simulink model "DYC_controller"  (R2018b)
settings: Solver=FixedStepAuto  StartTime=0.0  StopTime=inf  FixedStep=Ts  RelTol=1e-3  EnableMultiTasking=on
values from neighbouring files (symbols this model uses):
  A_vte = [1 0 -2*Ts*m_s/WB*(l_r*h_rc_f/w1+l_f*h_rc_r/w2) 0 -2*Ts*(K_f/w1+K_r/w2) ... (first row only)    [main.m]
  A_vte_p2 = [1 0 0 0 0 -Ts * m * hc / 2 / WB 0 -Ts * l_r * m * hc / WB / w1 ... (first row only)    [main.m]
  b1 = ones(4,1)/R    [main.m]
  boundary = 3000    [main.m]
  C_vte = [0 1 0 g 0 ... (first row only)    [main.m]
  C_vte_p2 = [1, -1, 1, -1, 0, 0, 0, 0 ... (first row only)    [main.m]
  eta = 0    [main.m]
  F_z1_s = l_r * m * g / 2 / WB    (= 9.45353456158)    [main.m]
  F_z2_s = F_z1_s    (= 9.45353456158)    [main.m]
  F_z3_s = l_f * m * g / 2 / WB    (= 9.11094809852)    [main.m]
  F_z4_s = F_z3_s    (= 9.11094809852)    [main.m]
  g = 9.81    [main.m]
  h_rc_f = 0.00    (= 0)    [main.m]
  h_rc_r = 0.00    (= 0)    [main.m]
  hc = 0.0751    [main.m]
  J = 0.9    [main.m]
  k1 = 2000    [main.m]
  k2 = 1000    [main.m]
  K_f = K_lin*l_cs^2*cos(phi*pi/180)    [main.m]
  K_r = K_lin*l_cs^2*cos(phi*pi/180)    [main.m]
  Kd = 0    [main.m]
  Ki = 75    [main.m]
  Kp = 600    [main.m]
  l_f = 0.1968    [main.m]
  l_r = 0.2042    [main.m]
  m = 3.832    [main.m]
  m_s = 0.9*m    (= 3.4488)    [main.m]
  mu = 0.8    [main.m]
  Protean_PD18_motormap = [2.92104016907 601.978033502 650.789692516 685.109940533 725.756581133 754.659963437 780.850883334 807.9513301 837.761936672 868.484372712 893.788791739 922.70944354 ... (50 elements, 25x2)]    [Protean_PD18_motormap.mat]
  Q_lat_process = 1E0*[var_r^2  0 0 0 0 0 0 0 0 ... (first row only)    [main.m]
  Q_lat_sensor = 1E-2*[var_r_s^2 0 0 0 ... (first row only)    [main.m]
  Q_meas_susp_p1 = [var_ay_m_p^2 0 0 0 ... (first row only)    [main.m]
  Q_meas_susp_p2 = [var_del_Fz^2 0 0 0 0 ... (first row only)    [main.m]
  R = 0.055    [main.m]
  Ts = 0.015    [main.m]
  V_x0 = (1000/3600)*V_x0    (= 11.1111111111)    [main.m]
  w1 = 0.2824    [main.m]
  w2 = 2.929    [main.m]
  WB = 0.406    [main.m]
undefined symbols (not defined in the file or in its folder): C_lf, C_lr, DiscIntNeverNeededParam, Discrete, t_e, Time
libraries: raspberrypilib x24, hdlsllib x21, simulink x17, discretizing x2, ctrlSharedLib x2, sharedTrackingLibrary x1
(part 2 of 3)

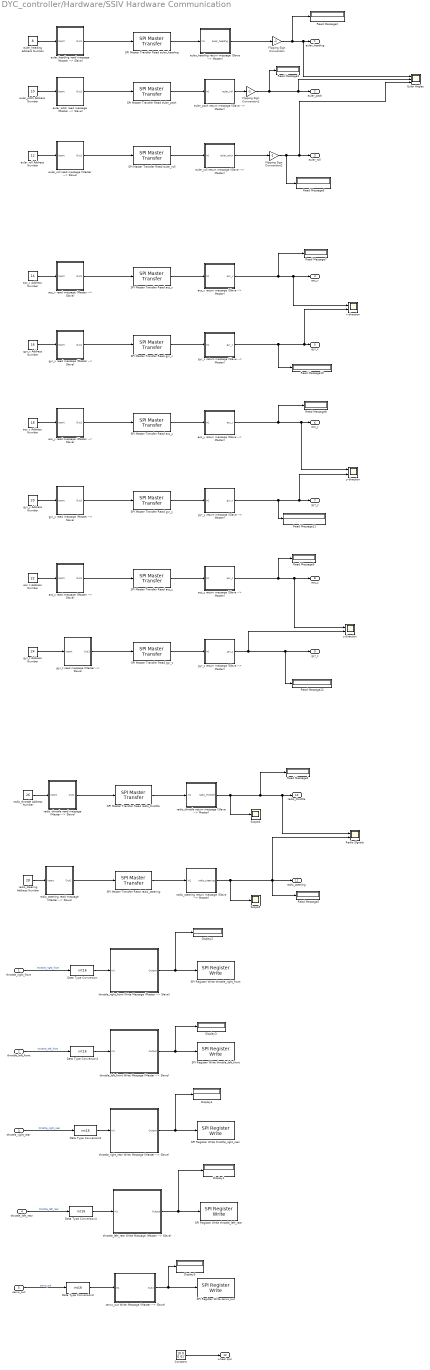
== system DYC_controller/Hardware/SSIV Hardware Communication ==
  throttle_right_front : Inport
  throttle_left_front : Inport  Port=2
  throttle_right_rear : Inport  Port=3
  throttle_left_rear : Inport  Port=4
  servo_out : Inport  Port=5
  Constant : Constant  Value=[0 0 0 0]'
  Data Type Conversion{,1..4} (5 alike) : DataTypeConversion  OutDataTypeStr=int16  RndMeth=Nearest
  Display{1..5} (5 alike) : Display
      settings: Format=decimal (Stored Integer)
  Euler Angles : Scope  NumInputPorts=3
  Flipping Sign Convention : Gain  Gain=-1
  Flipping Sign Convention1 : Gain  Gain=-1
  Flipping Sign Convention2 : Gain  Gain=-1
  Radio SIgnals : Scope  NumInputPorts=2
  Read Message{2..12} (11 alike) : Display
      settings: Format=decimal (Stored Integer)
  SPI Master Transfer Read acc_x : raspberrypilib/SPI Master Transfer  BoardProperty=Pi 3 Model B  SPIModule=uint32(0)  Mode=Master  BusSpeed=1000000  Pin=SPI0_CE1  FirstBitToTransfer=Most significant bit (MSB)  ClockMode=0  BlockFunction=Transfer  RegisterAddress=0  OutputDataType=int8  OutputDataLength=1
      settings: SourceProductName=Simulink Support Package for Raspberry Pi Hardware  SourceProductBaseCode=RASPPI
  SPI Master Transfer Read acc_y : raspberrypilib/SPI Master Transfer  BoardProperty=Pi 3 Model B  SPIModule=uint32(0)  Mode=Master  BusSpeed=1000000  Pin=SPI0_CE1  FirstBitToTransfer=Most significant bit (MSB)  ClockMode=0  BlockFunction=Transfer  RegisterAddress=0  OutputDataType=int8  OutputDataLength=1
      settings: SourceProductName=Simulink Support Package for Raspberry Pi Hardware  SourceProductBaseCode=RASPPI
  SPI Master Transfer Read acc_z : raspberrypilib/SPI Master Transfer  BoardProperty=Pi 3 Model B  SPIModule=uint32(0)  Mode=Master  BusSpeed=1000000  Pin=SPI0_CE1  FirstBitToTransfer=Most significant bit (MSB)  ClockMode=0  BlockFunction=Transfer  RegisterAddress=0  OutputDataType=int8  OutputDataLength=1
      settings: SourceProductName=Simulink Support Package for Raspberry Pi Hardware  SourceProductBaseCode=RASPPI
  SPI Master Transfer Read euler_heading : raspberrypilib/SPI Master Transfer  BoardProperty=Pi 3 Model B  SPIModule=uint32(0)  Mode=Master  BusSpeed=1000000  Pin=SPI0_CE1  FirstBitToTransfer=Most significant bit (MSB)  ClockMode=0  BlockFunction=Transfer  RegisterAddress=0  OutputDataType=int8  OutputDataLength=1
      settings: SourceProductName=Simulink Support Package for Raspberry Pi Hardware  SourceProductBaseCode=RASPPI
  SPI Master Transfer Read euler_pitch : raspberrypilib/SPI Master Transfer  BoardProperty=Pi 3 Model B  SPIModule=uint32(0)  Mode=Master  BusSpeed=1000000  Pin=SPI0_CE1  FirstBitToTransfer=Most significant bit (MSB)  ClockMode=0  BlockFunction=Transfer  RegisterAddress=0  OutputDataType=int8  OutputDataLength=1
      settings: SourceProductName=Simulink Support Package for Raspberry Pi Hardware  SourceProductBaseCode=RASPPI
  SPI Master Transfer Read euler_roll : raspberrypilib/SPI Master Transfer  BoardProperty=Pi 3 Model B  SPIModule=uint32(0)  Mode=Master  BusSpeed=1000000  Pin=SPI0_CE1  FirstBitToTransfer=Most significant bit (MSB)  ClockMode=0  BlockFunction=Transfer  RegisterAddress=0  OutputDataType=int8  OutputDataLength=1
      settings: SourceProductName=Simulink Support Package for Raspberry Pi Hardware  SourceProductBaseCode=RASPPI
  SPI Master Transfer Read gyr_x : raspberrypilib/SPI Master Transfer  BoardProperty=Pi 3 Model B  SPIModule=uint32(0)  Mode=Master  BusSpeed=1000000  Pin=SPI0_CE1  FirstBitToTransfer=Most significant bit (MSB)  ClockMode=0  BlockFunction=Transfer  RegisterAddress=0  OutputDataType=int8  OutputDataLength=1
      settings: SourceProductName=Simulink Support Package for Raspberry Pi Hardware  SourceProductBaseCode=RASPPI
  SPI Master Transfer Read gyr_y : raspberrypilib/SPI Master Transfer  BoardProperty=Pi 3 Model B  SPIModule=uint32(0)  Mode=Master  BusSpeed=1000000  Pin=SPI0_CE1  FirstBitToTransfer=Most significant bit (MSB)  ClockMode=0  BlockFunction=Transfer  RegisterAddress=0  OutputDataType=int8  OutputDataLength=1
      settings: SourceProductName=Simulink Support Package for Raspberry Pi Hardware  SourceProductBaseCode=RASPPI
  SPI Master Transfer Read gyr_z : raspberrypilib/SPI Master Transfer  BoardProperty=Pi 3 Model B  SPIModule=uint32(0)  Mode=Master  BusSpeed=1000000  Pin=SPI0_CE1  FirstBitToTransfer=Most significant bit (MSB)  ClockMode=0  BlockFunction=Transfer  RegisterAddress=0  OutputDataType=int8  OutputDataLength=1
      settings: SourceProductName=Simulink Support Package for Raspberry Pi Hardware  SourceProductBaseCode=RASPPI
  SPI Master Transfer Read radio_steering : raspberrypilib/SPI Master Transfer  BoardProperty=Pi 3 Model B  SPIModule=uint32(0)  Mode=Master  BusSpeed=1000000  Pin=SPI0_CE1  FirstBitToTransfer=Most significant bit (MSB)  ClockMode=0  BlockFunction=Transfer  RegisterAddress=0  OutputDataType=int8  OutputDataLength=1
      settings: SourceProductName=Simulink Support Package for Raspberry Pi Hardware  SourceProductBaseCode=RASPPI
  SPI Master Transfer Read radio_throttle : raspberrypilib/SPI Master Transfer  BoardProperty=Pi 3 Model B  SPIModule=uint32(0)  Mode=Master  BusSpeed=1000000  Pin=SPI0_CE1  FirstBitToTransfer=Most significant bit (MSB)  ClockMode=0  BlockFunction=Transfer  RegisterAddress=0  OutputDataType=int8  OutputDataLength=1
      settings: SourceProductName=Simulink Support Package for Raspberry Pi Hardware  SourceProductBaseCode=RASPPI
  "SPI Register Write servo_out " : raspberrypilib/SPI Register Write  BoardProperty=Pi 3 Model B  SPIModule=uint32(0)  Mode=Master  BusSpeed=1000000  Pin=SPI0_CE1  FirstBitToTransfer=Most significant bit (MSB)  ClockMode=0  BlockFunction=Write  RegisterAddress=38  OutputDataType=int8  OutputDataLength=1
      settings: SourceProductName=Simulink Support Package for Raspberry Pi Hardware  SourceProductBaseCode=RASPPI
  SPI Register Write throttle_left_front : raspberrypilib/SPI Register Write  BoardProperty=Pi 3 Model B  SPIModule=uint32(0)  Mode=Master  BusSpeed=1000000  Pin=SPI0_CE1  FirstBitToTransfer=Most significant bit (MSB)  ClockMode=0  BlockFunction=Write  RegisterAddress=32  OutputDataType=int8  OutputDataLength=1
      settings: SourceProductName=Simulink Support Package for Raspberry Pi Hardware  SourceProductBaseCode=RASPPI
  SPI Register Write throttle_left_rear : raspberrypilib/SPI Register Write  BoardProperty=Pi 3 Model B  SPIModule=uint32(0)  Mode=Master  BusSpeed=1000000  Pin=SPI0_CE1  FirstBitToTransfer=Most significant bit (MSB)  ClockMode=0  BlockFunction=Write  RegisterAddress=36  OutputDataType=int8  OutputDataLength=1
      settings: SourceProductName=Simulink Support Package for Raspberry Pi Hardware  SourceProductBaseCode=RASPPI
  SPI Register Write throttle_right_front : raspberrypilib/SPI Register Write  BoardProperty=Pi 3 Model B  SPIModule=uint32(0)  Mode=Master  BusSpeed=1000000  Pin=SPI0_CE1  FirstBitToTransfer=Most significant bit (MSB)  ClockMode=0  BlockFunction=Write  RegisterAddress=30  OutputDataType=int8  OutputDataLength=1
      settings: SourceProductName=Simulink Support Package for Raspberry Pi Hardware  SourceProductBaseCode=RASPPI
  SPI Register Write throttle_right_rear : raspberrypilib/SPI Register Write  BoardProperty=Pi 3 Model B  SPIModule=uint32(0)  Mode=Master  BusSpeed=1000000  Pin=SPI0_CE1  FirstBitToTransfer=Most significant bit (MSB)  ClockMode=0  BlockFunction=Write  RegisterAddress=34  OutputDataType=int8  OutputDataLength=1
      settings: SourceProductName=Simulink Support Package for Raspberry Pi Hardware  SourceProductBaseCode=RASPPI
  Scope4 : Scope
  Scope5 : Scope
  acc_x Address Number : Constant  Value=14  OutDataTypeStr=uint8
  acc_x read message (Master --> Slave) : Subsystem
  acc_x return message (Slave --> Master) : Subsystem
  acc_y Address Number : Constant  Value=18  OutDataTypeStr=uint8
  acc_y read message (Master --> Slave) : Subsystem
  acc_y return message (Slave --> Master) : Subsystem
  acc_z Address Number : Constant  Value=22  OutDataTypeStr=uint8
  acc_z read message (Master --> Slave) : Subsystem
  acc_z return message (Slave --> Master) : Subsystem
  euler_heading Address Number : Constant  Value=8  OutDataTypeStr=uint8
  euler_heading read message (Master --> Slave) : Subsystem
  euler_heading return message (Slave --> Master) : Subsystem
  euler_pitch Address Number : Constant  Value=10  OutDataTypeStr=uint8
  euler_pitch read message (Master --> Slave) : Subsystem
  euler_pitch return message (Slave --> Master) : Subsystem
  euler_roll Address Number : Constant  Value=12  OutDataTypeStr=uint8
  euler_roll read message (Master --> Slave) : Subsystem
  euler_roll return message (Slave --> Master) : Subsystem
  gyr_x Address Number : Constant  Value=16  OutDataTypeStr=uint8
  gyr_x read message (Master --> Slave) : Subsystem
  gyr_x return message (Slave --> Master) : Subsystem
  "gyr_y Address Number " : Constant  Value=20  OutDataTypeStr=uint8
  gyr_y read message (Master --> Slave) : Subsystem
  gyr_y return message (Slave --> Master) : Subsystem
  gyr_z Address Number : Constant  Value=24  OutDataTypeStr=uint8
  gyr_z read message (Master --> Slave) : Subsystem
  gyr_z return message (Slave --> Master) : Subsystem
  radio_steering Address Number : Constant  Value=28  OutDataTypeStr=uint8
  radio_steering read message (Master --> Slave) : Subsystem
  radio_steering return message (Slave --> Master) : Subsystem
  "radio_throttle Address Number " : Constant  Value=26  OutDataTypeStr=uint8
  radio_throttle read message (Master --> Slave) : Subsystem
  radio_throttle return message (Slave --> Master) : Subsystem
  servo_out Write Message (Master --> Slave) : Subsystem
  throttle_left_front Write Message (Master --> Slave) : Subsystem
  throttle_left_rear Write Message (Master --> Slave) : Subsystem
  throttle_right_front Write Message (Master --> Slave) : Subsystem
  throttle_right_rear Write Message (Master --> Slave) : Subsystem
  x-direction : Scope  NumInputPorts=2
  y-direction : Scope  NumInputPorts=2
  z-direction : Scope  NumInputPorts=2
  euler_heading : Outport
  euler_pitch : Outport  Port=2
  euler_roll : Outport  Port=3
  acc_x : Outport  Port=4
  gyr_x : Outport  Port=5
  acc_y : Outport  Port=6
  gyr_y : Outport  Port=7
  acc_z : Outport  Port=8
  gyr_z : Outport  Port=9
  radio_throttle : Outport  Port=10
  radio_steering : Outport  Port=11
  wheel spin : Outport  Port=12
  wires:
  euler_heading read message (Master --> Slave)/1(Out1) -> SPI Master Transfer Read euler_heading/1
  euler_heading return message (Slave --> Master)/1(euler_heading) -> Flipping Sign Convention/1
  SPI Master Transfer Read euler_heading/1 -> euler_heading return message (Slave --> Master)/1(In1)
  throttle_left_rear Write Message (Master --> Slave)/1(Output) -> Display1/1, SPI Register Write throttle_left_rear/1
  throttle_left_rear/1 -> Data Type Conversion4/1  "throttle_left_rear"
  SPI Master Transfer Read radio_throttle/1 -> radio_throttle return message (Slave --> Master)/1(In1)
  radio_throttle read message (Master --> Slave)/1(Out1) -> SPI Master Transfer Read radio_throttle/1
  radio_throttle return message (Slave --> Master)/1(radio_throttle) -> Read Message4/1, Radio SIgnals/1, radio_throttle/1, Scope4/1
  radio_steering return message (Slave --> Master)/1(radio_steering) -> radio_steering/1, Read Message5/1, Radio SIgnals/2, Scope5/1
  radio_steering read message (Master --> Slave)/1(Out1) -> SPI Master Transfer Read radio_steering/1
  SPI Master Transfer Read radio_steering/1 -> radio_steering return message (Slave --> Master)/1(In1)
  servo_out/1 -> Data Type Conversion3/1  "servo_out"
  servo_out Write Message (Master --> Slave)/1(Out1) -> Display5/1, "SPI Register Write servo_out "/1
  acc_x return message (Slave --> Master)/1(acc_x) -> Read Message7/1, x-direction/1, acc_x/1
  SPI Master Transfer Read acc_x/1 -> acc_x return message (Slave --> Master)/1(In1)
  acc_x read message (Master --> Slave)/1(Out1) -> SPI Master Transfer Read acc_x/1
  acc_y read message (Master --> Slave)/1(Out1) -> SPI Master Transfer Read acc_y/1
  SPI Master Transfer Read acc_y/1 -> acc_y return message (Slave --> Master)/1(In1)
  acc_y return message (Slave --> Master)/1(acc_y) -> y-direction/1, acc_y/1, Read Message8/1
  acc_z return message (Slave --> Master)/1(acc_z) -> z-direction/1, acc_z/1, Read Message9/1
  SPI Master Transfer Read acc_z/1 -> acc_z return message (Slave --> Master)/1(In1)
  acc_z read message (Master --> Slave)/1(Out1) -> SPI Master Transfer Read acc_z/1
  gyr_z read message (Master --> Slave)/1(Out1) -> SPI Master Transfer Read gyr_z/1
  SPI Master Transfer Read gyr_z/1 -> gyr_z return message (Slave --> Master)/1(In1)
  gyr_z return message (Slave --> Master)/1(gyr_z) -> z-direction/2, gyr_z/1, Read Message12/1
  gyr_y return message (Slave --> Master)/1(gyr_y) -> Read Message11/1, y-direction/2, gyr_y/1
  SPI Master Transfer Read gyr_y/1 -> gyr_y return message (Slave --> Master)/1(In1)
  gyr_y read message (Master --> Slave)/1(Out1) -> SPI Master Transfer Read gyr_y/1
  gyr_x read message (Master --> Slave)/1(Out1) -> SPI Master Transfer Read gyr_x/1
  SPI Master Transfer Read gyr_x/1 -> gyr_x return message (Slave --> Master)/1(In1)
  gyr_x return message (Slave --> Master)/1(gyr_x) -> x-direction/2, gyr_x/1, Read Message10/1
  throttle_right_front/1 -> Data Type Conversion/1  "throttle_right_front"
  throttle_right_front Write Message (Master --> Slave)/1(Output) -> SPI Register Write throttle_right_front/1, Display2/1
  throttle_right_rear Write Message (Master --> Slave)/1(Output) -> Display4/1, SPI Register Write throttle_right_rear/1
  throttle_right_rear/1 -> Data Type Conversion2/1  "throttle_right_rear"
  throttle_left_front/1 -> Data Type Conversion1/1  "throttle_left_front"
  throttle_left_front Write Message (Master --> Slave)/1(Output) -> SPI Register Write throttle_left_front/1, Display3/1
  Data Type Conversion/1 -> throttle_right_front Write Message (Master --> Slave)/1(In1)
  Data Type Conversion1/1 -> throttle_left_front Write Message (Master --> Slave)/1(In1)
  Data Type Conversion2/1 -> throttle_right_rear Write Message (Master --> Slave)/1(In1)
  Data Type Conversion3/1 -> servo_out Write Message (Master --> Slave)/1(In1)
  Data Type Conversion4/1 -> throttle_left_rear Write Message (Master --> Slave)/1(In1)
  "radio_throttle Address Number "/1 -> radio_throttle read message (Master --> Slave)/1(Inport)
  gyr_z Address Number/1 -> gyr_z read message (Master --> Slave)/1(Inport)
  "gyr_y Address Number "/1 -> gyr_y read message (Master --> Slave)/1(Inport)
  gyr_x Address Number/1 -> gyr_x read message (Master --> Slave)/1(Inport)
  acc_z Address Number/1 -> acc_z read message (Master --> Slave)/1(Inport)
  acc_y Address Number/1 -> acc_y read message (Master --> Slave)/1(Inport)
  acc_x Address Number/1 -> acc_x read message (Master --> Slave)/1(Inport)
  euler_heading Address Number/1 -> euler_heading read message (Master --> Slave)/1(Inport)
  radio_steering Address Number/1 -> radio_steering read message (Master --> Slave)/1(Inport)
  SPI Master Transfer Read euler_pitch/1 -> euler_pitch return message (Slave --> Master)/1(In1)
  euler_pitch Address Number/1 -> euler_pitch read message (Master --> Slave)/1(Inport)
  euler_pitch read message (Master --> Slave)/1(Out1) -> SPI Master Transfer Read euler_pitch/1
  euler_pitch return message (Slave --> Master)/1(euler_roll) -> Flipping Sign Convention1/1
  euler_roll return message (Slave --> Master)/1(euler_pitch) -> Flipping Sign Convention2/1
  euler_roll Address Number/1 -> euler_roll read message (Master --> Slave)/1(Inport)
  SPI Master Transfer Read euler_roll/1 -> euler_roll return message (Slave --> Master)/1(In1)
  euler_roll read message (Master --> Slave)/1(Out1) -> SPI Master Transfer Read euler_roll/1
  Flipping Sign Convention/1 -> Read Message2/1, Euler Angles/1, euler_heading/1
  Flipping Sign Convention1/1 -> Read Message3/1, Euler Angles/2, euler_pitch/1
  Flipping Sign Convention2/1 -> Read Message6/1, Euler Angles/3, euler_roll/1
  Constant/1 -> wheel spin/1

== system DYC_controller/Hardware/Throttle and Steering Handler ==
  note: MANUAL MODE THROTTLE
  note: DEAD SWITCH
  note: Note: If simulink loses connection (battery powered off) before the model is stopped, Simulink will freeze
  note: Can have the holding down the trigger as a condition for leaving the initialization code. THEN if the trigger is ever released, the code will stop running...may not want this after all, perhaps not for controllers without any integral action
  throttle : Inport
  Inport2 : Inport  Port=2
  steering angle : Inport  Port=3
  " " : Constant  Value=0
  Constant : Constant  Commented=on  Value=72
  Dead Switch : Switch  Threshold=-250
  Dead Switch Value : Constant  Value=200
  Gain : Gain  Gain=400/30
  Gain1 : Gain  Gain=180/pi
  Memory : Memory  Commented=on
  Relational Operator : RelationalOperator  RndMeth=Simplest
  Small Dead Zone For Safety : DeadZone  Commented=on  LowerValue=-10  UpperValue=10
  Stop Simulation : Stop  Commented=on
  Sum : Sum  Commented=on  Inputs=|+-
  Throttle RF : Outport
  Throttle LF : Outport  Port=2
  Throttle RR : Outport  Port=3
  Throttle LR : Outport  Port=4
  Outport : Outport  Port=5
  wires:
  " "/1 -> Dead Switch/3
  Inport2/1 -> Dead Switch/1
  Relational Operator/1 -> Dead Switch/2
  Dead Switch/1 -> Throttle LF/1, Throttle LR/1, Throttle RR/1, Throttle RF/1
  throttle/1 -> Relational Operator/1  "Throttle"
  Memory/1 -> Stop Simulation/1
  Dead Switch Value/1 -> Relational Operator/2
  Constant/1 -> Sum/2
  Sum/1 -> Small Dead Zone For Safety/1
  steering angle/1 -> Gain1/1  "[rad]"
  Gain/1 -> Outport/1  "[count]"
  Gain1/1 -> Gain/1  "[deg]"

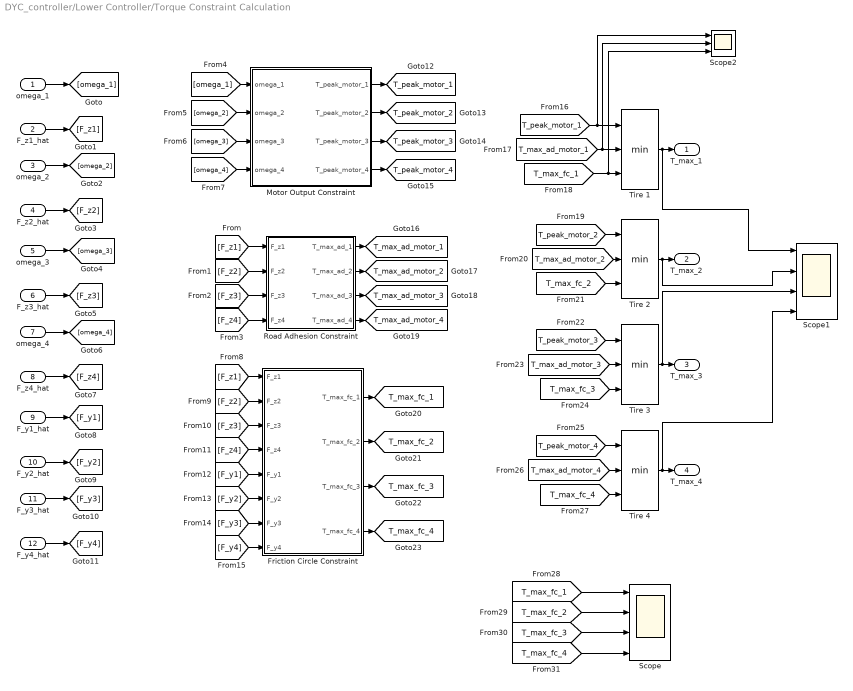
== system DYC_controller/Lower Controller/Torque Constraint Calculation ==
  omega_1 : Inport
  F_z1_hat : Inport  Port=2
  omega_2 : Inport  Port=3
  F_z2_hat : Inport  Port=4
  omega_3 : Inport  Port=5
  F_z3_hat : Inport  Port=6
  omega_4 : Inport  Port=7
  F_z4_hat : Inport  Port=8
  F_y1_hat : Inport  Port=9
  F_y2_hat : Inport  Port=10
  F_y3_hat : Inport  Port=11
  F_y4_hat : Inport  Port=12
  Friction Circle Constraint : Subsystem
  Motor Output Constraint : Subsystem
  Road Adhesion Constraint : Subsystem
  Scope : Scope  NumInputPorts=4
  Scope1 : Scope  NumInputPorts=4
  Scope2 : Scope  NumInputPorts=3
  Tire {1..4} (4 alike) : MinMax  Inputs=3
  T_max_1 : Outport
  T_max_2 : Outport  Port=2
  T_max_3 : Outport  Port=3
  T_max_4 : Outport  Port=4
  tag scope: T_max_ad_motor_1=global, T_max_ad_motor_2=global, T_max_ad_motor_3=global, T_max_ad_motor_4=global, T_max_fc_1=global, T_max_fc_2=global, T_max_fc_3=global, T_max_fc_4=global, T_peak_motor_1=global, T_peak_motor_2=global, T_peak_motor_3=global, T_peak_motor_4=global
  wires:
  omega_1/1 -> [omega_1]
  F_z1_hat/1 -> [F_z1]
  omega_2/1 -> [omega_2]
  F_z2_hat/1 -> [F_z2]
  F_z3_hat/1 -> [F_z3]
  omega_4/1 -> [omega_4]
  F_z4_hat/1 -> [F_z4]
  omega_3/1 -> [omega_3]
  [F_z1] -> Road Adhesion Constraint/1(F_z1)
  [F_z2] -> Road Adhesion Constraint/2(F_z2)
  [F_z3] -> Road Adhesion Constraint/3(F_z3)
  [F_z4] -> Road Adhesion Constraint/4(F_z4)
  [omega_1] -> Motor Output Constraint/1(omega_1)
  [omega_2] -> Motor Output Constraint/2(omega_2)
  [omega_3] -> Motor Output Constraint/3(omega_3)
  [omega_4] -> Motor Output Constraint/4(omega_4)
  F_y1_hat/1 -> [F_y1]
  F_y4_hat/1 -> [F_y4]
  F_y3_hat/1 -> [F_y3]
  F_y2_hat/1 -> [F_y2]
  [F_z1] -> Friction Circle Constraint/1(F_z1)
  [F_z2] -> Friction Circle Constraint/2(F_z2)
  [F_z3] -> Friction Circle Constraint/3(F_z3)
  [F_z4] -> Friction Circle Constraint/4(F_z4)
  [F_y1] -> Friction Circle Constraint/5(F_y1)
  [F_y2] -> Friction Circle Constraint/6(F_y2)
  [F_y3] -> Friction Circle Constraint/7(F_y3)
  [F_y4] -> Friction Circle Constraint/8(F_y4)
  Motor Output Constraint/1(T_peak_motor_1) -> [T_peak_motor_1]
  Motor Output Constraint/2(T_peak_motor_2) -> [T_peak_motor_2]
  Motor Output Constraint/3(T_peak_motor_3) -> [T_peak_motor_3]
  Motor Output Constraint/4(T_peak_motor_4) -> [T_peak_motor_4]
  Road Adhesion Constraint/1(T_max_ad_1) -> [T_max_ad_motor_1]
  Road Adhesion Constraint/2(T_max_ad_2) -> [T_max_ad_motor_2]
  Road Adhesion Constraint/3(T_max_ad_3) -> [T_max_ad_motor_3]
  Road Adhesion Constraint/4(T_max_ad_4) -> [T_max_ad_motor_4]
  Friction Circle Constraint/1(T_max_fc_1) -> [T_max_fc_1]
  Friction Circle Constraint/2(T_max_fc_2) -> [T_max_fc_2]
  Friction Circle Constraint/4(T_max_fc_4) -> [T_max_fc_4]
  [T_peak_motor_1] -> Tire 1/1, Scope2/1
  [T_max_ad_motor_1] -> Tire 1/2, Scope2/2
  [T_max_fc_1] -> Scope2/3, Tire 1/3
  [T_peak_motor_2] -> Tire 2/1
  [T_max_ad_motor_2] -> Tire 2/2
  [T_max_fc_2] -> Tire 2/3
  [T_peak_motor_3] -> Tire 3/1
  [T_max_ad_motor_3] -> Tire 3/2
  [T_max_fc_3] -> Tire 3/3
  [T_max_fc_4] -> Tire 4/3
  [T_max_ad_motor_4] -> Tire 4/2
  [T_peak_motor_4] -> Tire 4/1
  Tire 1/1 -> Scope1/1, T_max_1/1
  Tire 2/1 -> Scope1/2, T_max_2/1
  Tire 3/1 -> Scope1/3, T_max_3/1
  Tire 4/1 -> Scope1/4, T_max_4/1
  [T_max_fc_1] -> Scope/1
  [T_max_fc_2] -> Scope/2
  [T_max_fc_3] -> Scope/3
  [T_max_fc_4] -> Scope/4
  Friction Circle Constraint/3(T_max_fc_3) -> [T_max_fc_3]

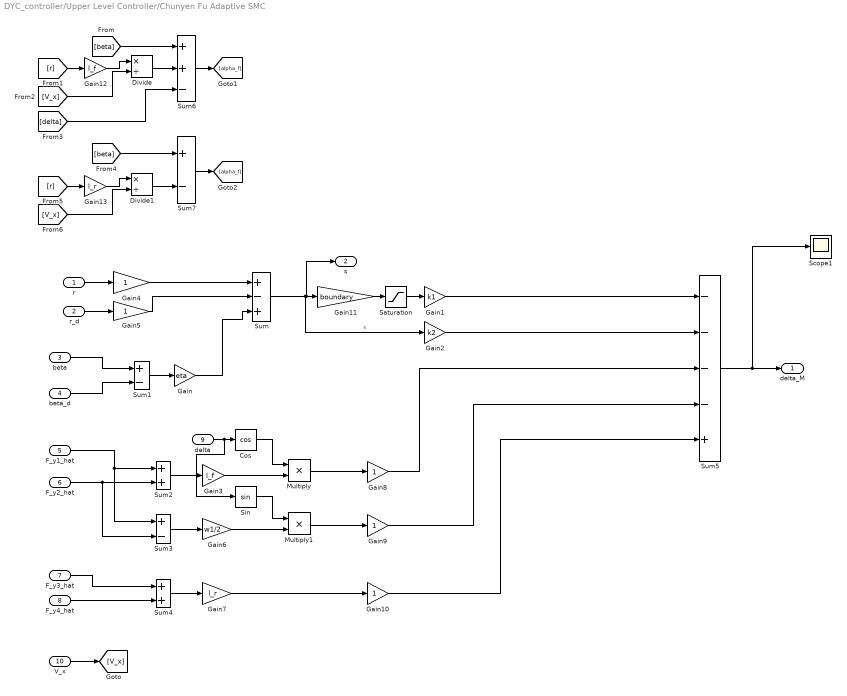
== system DYC_controller/Upper Level Controller/Chunyen Fu Adaptive SMC ==
  r : Inport
  r_d : Inport  Port=2
  beta : Inport  Port=3
  beta_d : Inport  Port=4
  F_y1_hat : Inport  Port=5
  F_y2_hat : Inport  Port=6
  F_y3_hat : Inport  Port=7
  F_y4_hat : Inport  Port=8
  delta : Inport  Port=9
  V_x : Inport  Port=10
  Cos : Trigonometry  Operator=cos
  Divide : Product  Inputs=*/
  Divide1 : Product  Inputs=*/
  Gain : Gain  Gain=eta
  Gain1 : Gain  Gain=k1
  Gain{4..5,8..10} (5 alike) : Gain
  Gain11 : Gain  Gain=boundary
  Gain12 : Gain  Gain=l_f
  Gain13 : Gain  Gain=l_r
  Gain2 : Gain  Gain=k2
  Gain3 : Gain  Gain=l_f
  Gain6 : Gain  Gain=w1/2
  Gain7 : Gain  Gain=l_r
  Multiply : Product
  Multiply1 : Product
  Saturation : Saturate  UpperLimit=1  LowerLimit=-1
  Scope1 : Scope
  Sin : Trigonometry
  Sum : Sum  Inputs=+-+
  Sum1 : Sum  Inputs=+-
  Sum2 : Sum
  Sum3 : Sum  Inputs=+-
  Sum4 : Sum
  Sum5 : Sum  Inputs=----+
  Sum6 : Sum  Inputs=++-
  Sum7 : Sum  Inputs=+-
  delta_M : Outport
  s : Outport  Port=2
  wires:
  beta_d/1 -> Sum1/2
  beta/1 -> Sum1/1
  r/1 -> Gain4/1
  r_d/1 -> Gain5/1
  Gain4/1 -> Sum/1
  Gain5/1 -> Sum/2
  Sum1/1 -> Gain/1
  Gain/1 -> Sum/3
  Sum/1 -> Gain2/1, s/1, Gain11/1  "s"
  Saturation/1 -> Gain1/1
  F_y2_hat/1 -> Sum3/2, Sum2/2
  Sum2/1 -> Gain3/1
  delta/1 -> Sin/1, Cos/1
  Gain3/1 -> Multiply/2
  Cos/1 -> Multiply/1
  F_y1_hat/1 -> Sum3/1, Sum2/1
  Sum3/1 -> Gain6/1
  Gain6/1 -> Multiply1/2
  Sin/1 -> Multiply1/1
  F_y3_hat/1 -> Sum4/1
  F_y4_hat/1 -> Sum4/2
  Sum4/1 -> Gain7/1
  Gain2/1 -> Sum5/2
  Gain7/1 -> Gain10/1
  Sum5/1 -> Scope1/1, delta_M/1
  Gain1/1 -> Sum5/1
  Gain8/1 -> Sum5/3
  Gain9/1 -> Sum5/4
  Gain10/1 -> Sum5/5
  Multiply1/1 -> Gain9/1
  Multiply/1 -> Gain8/1
  Gain11/1 -> Saturation/1
  [beta] -> Sum6/1
  [r] -> Gain12/1
  V_x/1 -> [V_x]
  Gain12/1 -> Divide/1
  Divide/1 -> Sum6/2
  [V_x] -> Divide/2
  [delta] -> Sum6/3
  Sum6/1 -> [alpha_f]
  Sum7/1 -> [alpha_f]
  [V_x] -> Divide1/2
  Divide1/1 -> Sum7/2
  Gain13/1 -> Divide1/1
  [r] -> Gain13/1
  [beta] -> Sum7/1

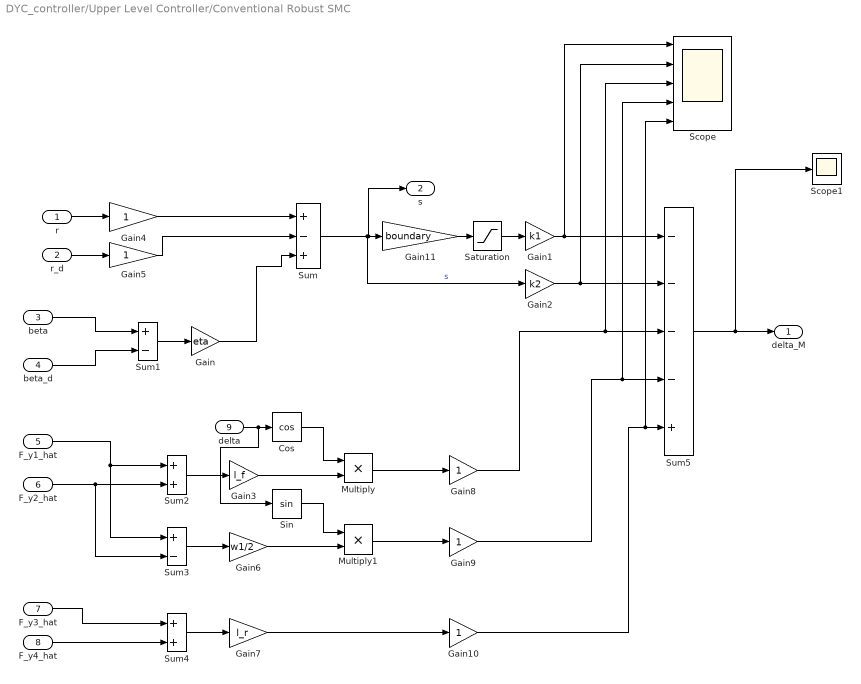
== system DYC_controller/Upper Level Controller/Conventional Robust SMC ==
  r : Inport
  r_d : Inport  Port=2
  beta : Inport  Port=3
  beta_d : Inport  Port=4
  F_y1_hat : Inport  Port=5
  F_y2_hat : Inport  Port=6
  F_y3_hat : Inport  Port=7
  F_y4_hat : Inport  Port=8
  delta : Inport  Port=9
  Cos : Trigonometry  Operator=cos
  Gain : Gain  Gain=eta
  Gain1 : Gain  Gain=k1
  Gain{4..5,8..10} (5 alike) : Gain
  Gain11 : Gain  Gain=boundary
  Gain2 : Gain  Gain=k2
  Gain3 : Gain  Gain=l_f
  Gain6 : Gain  Gain=w1/2
  Gain7 : Gain  Gain=l_r
  Multiply : Product
  Multiply1 : Product
  Saturation : Saturate  UpperLimit=1  LowerLimit=-1
  Scope : Scope  NumInputPorts=5
  Scope1 : Scope
  Sin : Trigonometry
  Sum : Sum  Inputs=+-+
  Sum1 : Sum  Inputs=+-
  Sum2 : Sum
  Sum3 : Sum  Inputs=+-
  Sum4 : Sum
  Sum5 : Sum  Inputs=----+
  delta_M : Outport
  s : Outport  Port=2
  wires:
  beta_d/1 -> Sum1/2
  beta/1 -> Sum1/1
  r/1 -> Gain4/1
  r_d/1 -> Gain5/1
  Gain4/1 -> Sum/1
  Gain5/1 -> Sum/2
  Sum1/1 -> Gain/1
  Gain/1 -> Sum/3
  Sum/1 -> Gain2/1, s/1, Gain11/1  "s"
  Saturation/1 -> Gain1/1
  F_y2_hat/1 -> Sum3/2, Sum2/2
  Sum2/1 -> Gain3/1
  delta/1 -> Sin/1, Cos/1
  Gain3/1 -> Multiply/2
  Cos/1 -> Multiply/1
  F_y1_hat/1 -> Sum3/1, Sum2/1
  Sum3/1 -> Gain6/1
  Gain6/1 -> Multiply1/2
  Sin/1 -> Multiply1/1
  F_y3_hat/1 -> Sum4/1
  F_y4_hat/1 -> Sum4/2
  Sum4/1 -> Gain7/1
  Gain2/1 -> Scope/2, Sum5/2
  Gain7/1 -> Gain10/1
  Sum5/1 -> Scope1/1, delta_M/1
  Gain1/1 -> Scope/1, Sum5/1
  Gain8/1 -> Scope/3, Sum5/3
  Gain9/1 -> Scope/4, Sum5/4
  Gain10/1 -> Scope/5, Sum5/5
  Multiply1/1 -> Gain9/1
  Multiply/1 -> Gain8/1
  Gain11/1 -> Saturation/1

== system DYC_controller/Upper Level Controller/Speed Controller ==
  speed error : Inport
  Discrete-Time Integrator : DiscreteIntegrator  SampleTime=-1  ICPrevOutput=DiscIntNeverNeededParam  ICPrevScaledInput=DiscIntNeverNeededParam
  Discrete-Time Integrator1 : DiscreteIntegrator  SampleTime=-1  ICPrevOutput=DiscIntNeverNeededParam  ICPrevScaledInput=DiscIntNeverNeededParam
  Gain : Gain  Gain=Kp
  Gain1 : Gain  Gain=Ki
  Gain2 : Gain  Gain=Kd
  Sum : Sum  Inputs=+++
  T_base : Outport
  wires:
  Sum/1 -> T_base/1
  speed error/1 -> Gain/1, Discrete-Time Integrator/1, Discrete-Time Integrator1/1
  Discrete-Time Integrator/1 -> Gain1/1
  Gain1/1 -> Sum/2
  Discrete-Time Integrator1/1 -> Gain2/1
  Gain2/1 -> Sum/3
  Gain/1 -> Sum/1

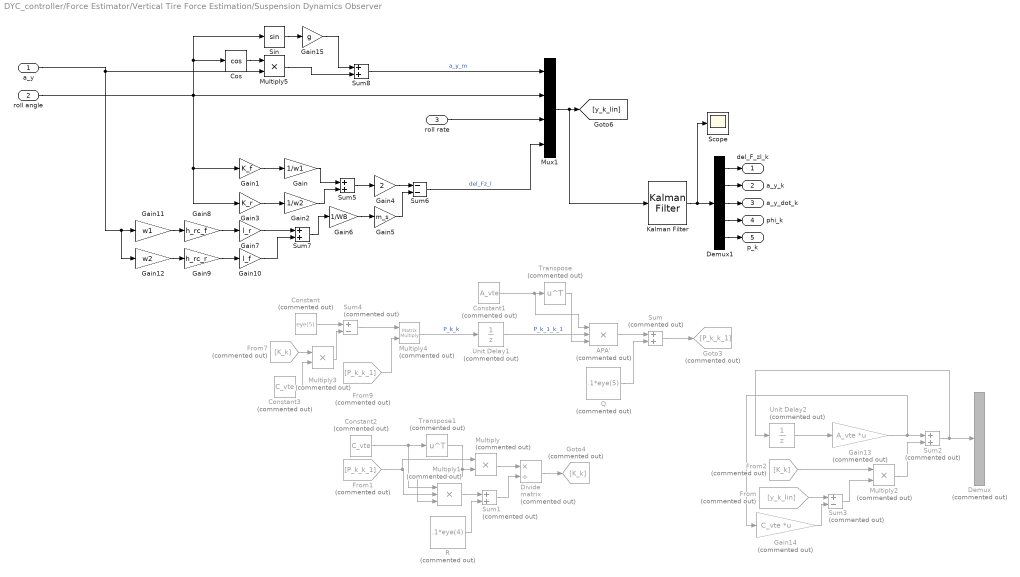
== system DYC_controller/Force Estimator/Vertical Tire Force Estimation/Suspension Dynamics Observer ==
  a_y : Inport
  roll angle : Inport  Port=2
  roll rate : Inport  Port=3
  APA' : Product  Commented=on  Inputs=3
  Constant : Constant  Commented=on  Value=eye(5)
  Constant1 : Constant  Commented=on  Value=A_vte
  Constant2 : Constant  Commented=on  Value=C_vte
  Constant3 : Constant  Commented=on  Value=C_vte
  Cos : Trigonometry  Operator=cos
  Demux : Demux  Commented=on  Outputs=5
  Demux1 : Demux  Outputs=5
  Divide : Product  Commented=on  Inputs=*/  Multiplication=Matrix(*)
  From : From  Commented=on  GotoTag=y_k_lin
  From1 : From  Commented=on  GotoTag=P_k_k_1
  From2 : From  Commented=on  GotoTag=K_k
  From7 : From  Commented=on  GotoTag=K_k
  From9 : From  Commented=on  GotoTag=P_k_k_1
  Gain : Gain  Gain=1/w1
  Gain1 : Gain  Gain=K_f
  Gain10 : Gain  Gain=l_f
  Gain11 : Gain  Gain=w1
  Gain12 : Gain  Gain=w2
  Gain13 : Gain  Commented=on  Gain=A_vte  Multiplication=Matrix(K*u) (u vector)
  Gain14 : Gain  Commented=on  Gain=C_vte  Multiplication=Matrix(K*u) (u vector)
  Gain15 : Gain  Gain=g
  Gain2 : Gain  Gain=1/w2
  Gain3 : Gain  Gain=K_r
  Gain4 : Gain  Gain=2
  Gain5 : Gain  Gain=m_s
  Gain6 : Gain  Gain=1/WB
  Gain7 : Gain  Gain=l_r
  Gain8 : Gain  Gain=h_rc_f
  Gain9 : Gain  Gain=h_rc_r
  Goto3 : Goto  Commented=on  GotoTag=P_k_k_1
  Goto4 : Goto  Commented=on  GotoTag=K_k
  Kalman Filter : ctrlSharedLib/Kalman Filter  TimeDomain=Discrete-Time  UseCurrentEstimator=on  ModelSource=Individual A, B, C, D matrices  ModelSourceVariable=ss(0.95,1,1,0,1)  A=A_vte  B=0  C=C_vte  D=0  NumberOfStates=1  NumberOfInputs=1  NumberOfOutputs=1  InitialEstimateSource=Dialog  X0=[0 0 0 0 0]'  P0=10  UseK=off  UseGH=off  NumberOfProcessNoiseInputs=1  G=1  TimeInvariantG=on  H=0  TimeInvariantH=on  Q=Q_proc_susp_p1  TimeInvariantQ=on  R=Q_meas_susp_p1  TimeInvariantR=on  N=0  TimeInvariantN=on  AddInputPort=off  AddEnablePort=off  OutputEstimatedY=off  OutputP=off  Ts=Ts
      settings: SourceProductBaseCode=CT
  Multiply : Product  Commented=on
  Multiply1 : Product  Commented=on  Inputs=3
  Multiply2 : Product  Commented=on
  Multiply3 : Product  Commented=on
  Multiply4 : Product  Commented=on  Multiplication=Matrix(*)
  Multiply5 : Product
  Mux1 : Mux
  Q : Constant  Commented=on  Value=.1*eye(5)
  R : Constant  Commented=on  Value=.1*eye(4)
  Scope : Scope
  Sin : Trigonometry
  Sum : Sum  Commented=on
  Sum1 : Sum  Commented=on
  Sum2 : Sum  Commented=on
  Sum3 : Sum  Commented=on  Inputs=+-
  Sum4 : Sum  Commented=on  Inputs=+-
  Sum5 : Sum
  Sum6 : Sum  Inputs=--
  Sum7 : Sum
  Sum8 : Sum
  Transpose : Math  Commented=on  Operator=transpose  SaturateOnIntegerOverflow=on
  Transpose1 : Math  Commented=on  Operator=transpose  SaturateOnIntegerOverflow=on
  Unit Delay1 : UnitDelay  Commented=on  InitialCondition=ones(5)  SampleTime=-1
  Unit Delay2 : UnitDelay  Commented=on  InitialCondition=[0; 0; 0; 0; 0]  SampleTime=-1
  del_F_zl_k : Outport
  a_y_k : Outport  Port=2
  a_y_dot_k : Outport  Port=3
  phi_k : Outport  Port=4
  p_k : Outport  Port=5
  wires:
  Gain10/1 -> Sum7/2
  Gain12/1 -> Gain9/1
  Gain4/1 -> Sum6/1
  Sum6/1 -> Mux1/4  "del_Fz_l"
  Sum5/1 -> Gain4/1
  Gain8/1 -> Gain7/1
  Gain2/1 -> Sum5/2
  Gain9/1 -> Gain10/1
  Gain3/1 -> Gain2/1
  Sum7/1 -> Gain6/1
  Gain1/1 -> Gain/1
  Gain/1 -> Sum5/1
  Gain7/1 -> Sum7/1
  Gain11/1 -> Gain8/1
  Gain6/1 -> Gain5/1
  Gain5/1 -> Sum6/2
  Constant3/1 -> Multiply3/2
  Sum4/1 -> Multiply4/1
  Constant/1 -> Sum4/1
  Sum/1 -> Goto3/1
  From7/1 -> Multiply3/1
  Transpose/1 -> APA'/3
  Q/1 -> Sum/2
  Constant1/1 -> APA'/1, Transpose/1
  Unit Delay1/1 -> APA'/2  "P_k_1_k_1"
  APA'/1 -> Sum/1
  Multiply4/1 -> Unit Delay1/1  "P_k_k"
  Multiply3/1 -> Sum4/2
  From9/1 -> Multiply4/2
  Sum1/1 -> Divide/2
  Constant2/1 -> Multiply1/1, Transpose1/1
  Multiply/1 -> Divide/1
  From1/1 -> Multiply/1, Multiply1/2
  Multiply1/1 -> Sum1/1
  R/1 -> Sum1/2
  Transpose1/1 -> Multiply/2, Multiply1/3
  Divide/1 -> Goto4/1
  Unit Delay2/1 -> Gain13/1
  Multiply2/1 -> Sum2/2
  Sum3/1 -> Multiply2/2
  From/1 -> Sum3/1
  Gain14/1 -> Sum3/2
  Gain13/1 -> Sum2/1, Gain14/1
  Sum2/1 -> Demux/1, Unit Delay2/1
  From2/1 -> Multiply2/1
  Cos/1 -> Multiply5/1
  Multiply5/1 -> Sum8/2
  Sin/1 -> Gain15/1
  Gain15/1 -> Sum8/1
  Sum8/1 -> Mux1/1  "a_y_m"
  roll angle/1 -> Mux1/2, Gain1/1, Gain3/1, Sin/1, Cos/1
  roll rate/1 -> Mux1/3
  a_y/1 -> Gain11/1, Gain12/1, Multiply5/2
  Demux1/3 -> a_y_dot_k/1
  Demux1/2 -> a_y_k/1
  Demux1/1 -> del_F_zl_k/1
  Demux1/5 -> p_k/1
  Kalman Filter/1 -> Scope/1, Demux1/1
  Demux1/4 -> phi_k/1
  Mux1/1 -> Kalman Filter/1, [y_k_lin]

== system DYC_controller/Hardware/SSIV Hardware Communication/acc_x read message (Master --> Slave) ==
  Inport : Inport
  Mux : Mux
      settings: DisplayOption=signals
  Read Bit Set : simulink/Logic and Bit Operations/Bit Set  iBit=7
      settings: SourceProductName=Simulink  SourceProductBaseCode=SL
  uint8_t 1 : Constant  OutDataTypeStr=uint8
  uint8_t 2 : Constant  OutDataTypeStr=uint8
  uint8_t 3 : Constant  OutDataTypeStr=uint8
  Out1 : Outport
  wires:
  Read Bit Set/1 -> Mux/1  "Addres/RW Byte acc_x Teensy Status will be returned here"
  uint8_t 1/1 -> Mux/2  "Junk will be returned here"
  Inport/1 -> Read Bit Set/1
  uint8_t 3/1 -> Mux/4  "Byte 1 will be returned here"
  Mux/1 -> Out1/1
  uint8_t 2/1 -> Mux/3  "Byte 0 will be returned here"

== system DYC_controller/Hardware/SSIV Hardware Communication/acc_x return message (Slave --> Master) ==
  In1 : Inport
  8 bytes concatinated converted to double : DataTypeConversion  OutDataTypeStr=double  RndMeth=Nearest
  Acceleration Int to Double Scale Factor : Gain  Gain=1/100
  Bit Concat : hdlsllib/Logic and Bit Operations/Bit Concat  numInputs=2
      settings: SourceProductName=HDL Coder  SourceProductBaseCode=HD
  Bytes of the return message : Display
      settings: Format=decimal (Stored Integer)
  Data Type Conversion : DataTypeConversion  OutDataTypeStr=int16  RndMeth=Nearest
  Demux : Demux
  Display : Display
      settings: Format=binary (Stored Integer)
  Display1 : Display
      settings: Format=decimal (Stored Integer)
  Display2 : Display
      settings: Format=binary (Stored Integer)
  acc_x : Outport
  wires:
  8 bytes concatinated converted to double/1 -> Acceleration Int to Double Scale Factor/1  "acc_x"
  Demux/2 -> Display2/1  "Slave Status"
  Demux/1 -> Display/1  "Previous Data"
  In1/1 -> Bytes of the return message/1, Demux/1
  Bit Concat/1 -> Data Type Conversion/1
  Demux/4 -> Bit Concat/1
  Demux/3 -> Bit Concat/2
  Acceleration Int to Double Scale Factor/1 -> Display1/1, acc_x/1
  Data Type Conversion/1 -> 8 bytes concatinated converted to double/1

== system DYC_controller/Hardware/SSIV Hardware Communication/acc_y read message (Master --> Slave) ==
  Inport : Inport
  Mux : Mux
      settings: DisplayOption=signals
  Read Bit Set : simulink/Logic and Bit Operations/Bit Set  iBit=7
      settings: SourceProductName=Simulink  SourceProductBaseCode=SL
  uint8_t 1 : Constant  OutDataTypeStr=uint8
  uint8_t 2 : Constant  OutDataTypeStr=uint8
  uint8_t 3 : Constant  OutDataTypeStr=uint8
  Out1 : Outport
  wires:
  uint8_t 2/1 -> Mux/3  "Byte 0 will be returned here"
  Mux/1 -> Out1/1
  uint8_t 3/1 -> Mux/4  "Byte 1 will be returned here"
  Inport/1 -> Read Bit Set/1
  uint8_t 1/1 -> Mux/2  "Junk will be returned here"
  Read Bit Set/1 -> Mux/1  "Addres/RW Byte acc_y Teensy Status will be returned here"

== system DYC_controller/Hardware/SSIV Hardware Communication/acc_y return message (Slave --> Master) ==
  In1 : Inport
  8 bytes concatinated converted to double : DataTypeConversion  OutDataTypeStr=double  RndMeth=Nearest
  Acceleration Int to Double Scale Factor : Gain  Gain=1/100
  Bit Concat : hdlsllib/Logic and Bit Operations/Bit Concat  numInputs=2
      settings: SourceProductName=HDL Coder  SourceProductBaseCode=HD
  Bytes of the return message : Display
      settings: Format=decimal (Stored Integer)
  Data Type Conversion : DataTypeConversion  OutDataTypeStr=int16  RndMeth=Nearest
  Demux : Demux
  Display : Display
      settings: Format=binary (Stored Integer)
  Display1 : Display
      settings: Format=decimal (Stored Integer)
  Display2 : Display
      settings: Format=binary (Stored Integer)
  acc_y : Outport
  wires:
  Acceleration Int to Double Scale Factor/1 -> acc_y/1, Display1/1
  Demux/3 -> Bit Concat/2
  Demux/4 -> Bit Concat/1
  Bit Concat/1 -> Data Type Conversion/1
  In1/1 -> Demux/1, Bytes of the return message/1
  Demux/1 -> Display/1  "Previous Data"
  Demux/2 -> Display2/1  "Slave Status"
  8 bytes concatinated converted to double/1 -> Acceleration Int to Double Scale Factor/1  "acc_y"
  Data Type Conversion/1 -> 8 bytes concatinated converted to double/1

== system DYC_controller/Hardware/SSIV Hardware Communication/acc_z read message (Master --> Slave) ==
  Inport : Inport
  Mux : Mux
      settings: DisplayOption=signals
  Read Bit Set : simulink/Logic and Bit Operations/Bit Set  iBit=7
      settings: SourceProductName=Simulink  SourceProductBaseCode=SL
  uint8_t 1 : Constant  OutDataTypeStr=uint8
  uint8_t 2 : Constant  OutDataTypeStr=uint8
  uint8_t 3 : Constant  OutDataTypeStr=uint8
  Out1 : Outport
  wires:
  Read Bit Set/1 -> Mux/1  "Addres/RW Byte acc_y Teensy Status will be returned here"
  uint8_t 1/1 -> Mux/2  "Junk will be returned here"
  Inport/1 -> Read Bit Set/1
  uint8_t 3/1 -> Mux/4  "Byte 1 will be returned here"
  Mux/1 -> Out1/1
  uint8_t 2/1 -> Mux/3  "Byte 0 will be returned here"

== system DYC_controller/Hardware/SSIV Hardware Communication/acc_z return message (Slave --> Master) ==
  In1 : Inport
  8 bytes concatinated converted to double : DataTypeConversion  OutDataTypeStr=double  RndMeth=Nearest
  Acceleration Int to Double Scale Factor : Gain  Gain=1/100
  Bit Concat : hdlsllib/Logic and Bit Operations/Bit Concat  numInputs=2
      settings: SourceProductName=HDL Coder  SourceProductBaseCode=HD
  Bytes of the return message : Display
      settings: Format=decimal (Stored Integer)
  Data Type Conversion : DataTypeConversion  OutDataTypeStr=int16  RndMeth=Nearest
  Demux : Demux
  Display : Display
      settings: Format=binary (Stored Integer)
  Display1 : Display
      settings: Format=decimal (Stored Integer)
  Display2 : Display
      settings: Format=binary (Stored Integer)
  acc_z : Outport
  wires:
  8 bytes concatinated converted to double/1 -> Acceleration Int to Double Scale Factor/1  "acc_z"
  Demux/2 -> Display2/1  "Slave Status"
  Demux/1 -> Display/1  "Previous Data"
  In1/1 -> Bytes of the return message/1, Demux/1
  Bit Concat/1 -> Data Type Conversion/1
  Demux/4 -> Bit Concat/1
  Demux/3 -> Bit Concat/2
  Acceleration Int to Double Scale Factor/1 -> Display1/1, acc_z/1
  Data Type Conversion/1 -> 8 bytes concatinated converted to double/1

== system DYC_controller/Hardware/SSIV Hardware Communication/euler_heading read message (Master --> Slave) ==
  Inport : Inport
  Mux : Mux
      settings: DisplayOption=signals
  Read Bit Set : simulink/Logic and Bit Operations/Bit Set  iBit=7
      settings: SourceProductName=Simulink  SourceProductBaseCode=SL
  uint8_t  1 : Constant  OutDataTypeStr=uint8
  uint8_t  2 : Constant  OutDataTypeStr=uint8
  uint8_t  3 : Constant  OutDataTypeStr=uint8
  Out1 : Outport
  wires:
  Read Bit Set/1 -> Mux/1  "Addres/RW Byte euler_heading Teensy Status will be returned here"
  Inport/1 -> Read Bit Set/1
  uint8_t  3/1 -> Mux/4  "Byte 1 will be returned here"
  Mux/1 -> Out1/1
  uint8_t  2/1 -> Mux/3  "Byte 0 will be returned here"
  uint8_t  1/1 -> Mux/2  "Junk will be returned here"

== system DYC_controller/Hardware/SSIV Hardware Communication/euler_heading return message (Slave --> Master) ==
  In1 : Inport
  Bit Concat : hdlsllib/Logic and Bit Operations/Bit Concat  numInputs=2
      settings: SourceProductName=HDL Coder  SourceProductBaseCode=HD
  Bytes of the return message : Display
      settings: Format=decimal (Stored Integer)
  Data Type Conversion : DataTypeConversion  OutDataTypeStr=int16  RndMeth=Nearest
  Demux : Demux
  Display : Display
      settings: Format=binary (Stored Integer)
  Display1 : Display
      settings: Format=decimal (Stored Integer)
  Display2 : Display
      settings: Format=binary (Stored Integer)
  Euler Int to Double Scale Factor : Gain  Gain=1/16
  Scope : Scope
  Scope1 : Scope
  concatinate bytes and convert to double : DataTypeConversion  OutDataTypeStr=double  RndMeth=Nearest  LockScale=on
  euler_heading : Outport
  wires:
  concatinate bytes and convert to double/1 -> Euler Int to Double Scale Factor/1
  Demux/2 -> Display2/1  "Slave Status"
  Demux/1 -> Display/1  "Previous Data"
  In1/1 -> Bytes of the return message/1, Scope1/1, Demux/1
  Demux/4 -> Bit Concat/1
  Demux/3 -> Bit Concat/2
  Euler Int to Double Scale Factor/1 -> Display1/1, euler_heading/1
  Bit Concat/1 -> Data Type Conversion/1
  Data Type Conversion/1 -> Scope/1, concatinate bytes and convert to double/1

== system DYC_controller/Hardware/SSIV Hardware Communication/euler_pitch read message (Master --> Slave) ==
  Inport : Inport
  Mux : Mux
      settings: DisplayOption=signals
  Read Bit Set : simulink/Logic and Bit Operations/Bit Set  iBit=7
      settings: SourceProductName=Simulink  SourceProductBaseCode=SL
  uint8_t  1 : Constant  OutDataTypeStr=uint8
  uint8_t  2 : Constant  OutDataTypeStr=uint8
  uint8_t  3 : Constant  OutDataTypeStr=uint8
  Out1 : Outport
  wires:
  Read Bit Set/1 -> Mux/1  "Addres/RW Byte euler_roll Teensy Status will be returned here"
  Inport/1 -> Read Bit Set/1
  uint8_t  3/1 -> Mux/4  "Byte 1 will be returned here"
  Mux/1 -> Out1/1
  uint8_t  2/1 -> Mux/3  "Byte 0 will be returned here"
  uint8_t  1/1 -> Mux/2  "Junk will be returned here"

== system DYC_controller/Hardware/SSIV Hardware Communication/euler_pitch return message (Slave --> Master) ==
  In1 : Inport
  8 bytes concatinated converted to double : DataTypeConversion  OutDataTypeStr=double  RndMeth=Nearest
  Bit Concat : hdlsllib/Logic and Bit Operations/Bit Concat  numInputs=2
      settings: SourceProductName=HDL Coder  SourceProductBaseCode=HD
  Bytes of the return message : Display
      settings: Format=decimal (Stored Integer)
  Data Type Conversion : DataTypeConversion  OutDataTypeStr=int16  RndMeth=Nearest
  Demux : Demux
  Display : Display
      settings: Format=binary (Stored Integer)
  Display1 : Display
      settings: Format=decimal (Stored Integer)
  Display2 : Display
      settings: Format=binary (Stored Integer)
  Euler Int to Double Scale Factor : Gain  Gain=1/16
  Scope : Scope
  euler_roll : Outport
  wires:
  8 bytes concatinated converted to double/1 -> Euler Int to Double Scale Factor/1
  Demux/2 -> Display2/1  "Slave Status"
  Demux/1 -> Display/1  "Previous Data"
  In1/1 -> Bytes of the return message/1, Demux/1
  Bit Concat/1 -> Data Type Conversion/1
  Demux/4 -> Bit Concat/1
  Demux/3 -> Bit Concat/2
  Euler Int to Double Scale Factor/1 -> Display1/1, euler_roll/1
  Data Type Conversion/1 -> Scope/1, 8 bytes concatinated converted to double/1

== system DYC_controller/Hardware/SSIV Hardware Communication/euler_roll read message (Master --> Slave) ==
  Inport : Inport
  Mux : Mux
      settings: DisplayOption=signals
  Read Bit Set : simulink/Logic and Bit Operations/Bit Set  iBit=7
      settings: SourceProductName=Simulink  SourceProductBaseCode=SL
  uint8_t 1 : Constant  OutDataTypeStr=uint8
  uint8_t 2 : Constant  OutDataTypeStr=uint8
  uint8_t 3 : Constant  OutDataTypeStr=uint8
  Out1 : Outport
  wires:
  Read Bit Set/1 -> Mux/1  "Addres/RW Byte euler_pitch Teensy Status will be returned here"
  uint8_t 1/1 -> Mux/2  "Junk will be returned here"
  Inport/1 -> Read Bit Set/1
  uint8_t 3/1 -> Mux/4  "Byte 1 will be returned here"
  Mux/1 -> Out1/1
  uint8_t 2/1 -> Mux/3  "Byte 0 will be returned here"

== system DYC_controller/Hardware/SSIV Hardware Communication/euler_roll return message (Slave --> Master) ==
  In1 : Inport
  8 bytes concatinated converted to double : DataTypeConversion  OutDataTypeStr=double  RndMeth=Nearest
  Bit Concat : hdlsllib/Logic and Bit Operations/Bit Concat  numInputs=2
      settings: SourceProductName=HDL Coder  SourceProductBaseCode=HD
  Bytes of the return message : Display
      settings: Format=decimal (Stored Integer)
  Data Type Conversion : DataTypeConversion  OutDataTypeStr=int16
  Demux : Demux
  Display : Display
      settings: Format=binary (Stored Integer)
  Display1 : Display
      settings: Format=decimal (Stored Integer)
  Display2 : Display
      settings: Format=binary (Stored Integer)
  Euler Int to Double Scale Factor : Gain  Gain=1/16  SaturateOnIntegerOverflow=on
  Scope : Scope
  euler_pitch : Outport
  wires:
  8 bytes concatinated converted to double/1 -> Euler Int to Double Scale Factor/1
  Demux/2 -> Display2/1  "Slave Status"
  Demux/1 -> Display/1  "Previous Data"
  In1/1 -> Bytes of the return message/1, Demux/1
  Bit Concat/1 -> Data Type Conversion/1
  Demux/4 -> Bit Concat/1
  Demux/3 -> Bit Concat/2
  Euler Int to Double Scale Factor/1 -> Display1/1, euler_pitch/1
  Data Type Conversion/1 -> Scope/1, 8 bytes concatinated converted to double/1

== system DYC_controller/Hardware/SSIV Hardware Communication/gyr_x read message (Master --> Slave) ==
  Inport : Inport
  Mux : Mux
      settings: DisplayOption=signals
  Read Bit Set : simulink/Logic and Bit Operations/Bit Set  iBit=7
      settings: SourceProductName=Simulink  SourceProductBaseCode=SL
  uint8_t 1 : Constant  OutDataTypeStr=uint8
  uint8_t 2 : Constant  OutDataTypeStr=uint8
  uint8_t 3 : Constant  OutDataTypeStr=uint8
  Out1 : Outport
  wires:
  uint8_t 2/1 -> Mux/3  "Byte 0 will be returned here"
  Mux/1 -> Out1/1
  uint8_t 3/1 -> Mux/4  "Byte 1 will be returned here"
  Inport/1 -> Read Bit Set/1
  uint8_t 1/1 -> Mux/2  "Junk will be returned here"
  Read Bit Set/1 -> Mux/1  "Addres/RW Byte gyr_x Teensy Status will be returned here"

== system DYC_controller/Hardware/SSIV Hardware Communication/gyr_x return message (Slave --> Master) ==
  In1 : Inport
  8 bytes concatinated converted to double : DataTypeConversion  OutDataTypeStr=double  RndMeth=Nearest
  Bit Concat : hdlsllib/Logic and Bit Operations/Bit Concat  numInputs=2
      settings: SourceProductName=HDL Coder  SourceProductBaseCode=HD
  Bytes of the return message : Display
      settings: Format=decimal (Stored Integer)
  Data Type Conversion : DataTypeConversion  OutDataTypeStr=int16  RndMeth=Nearest
  Demux : Demux
  Display : Display
      settings: Format=binary (Stored Integer)
  Display1 : Display
      settings: Format=decimal (Stored Integer)
  Display2 : Display
      settings: Format=binary (Stored Integer)
  Gyroscope Int to Double Scale Factor : Gain  Gain=1/900
  gyr_x : Outport
  wires:
  Gyroscope Int to Double Scale Factor/1 -> gyr_x/1, Display1/1
  Demux/3 -> Bit Concat/2
  Demux/4 -> Bit Concat/1
  Bit Concat/1 -> Data Type Conversion/1
  In1/1 -> Demux/1, Bytes of the return message/1
  Demux/1 -> Display/1  "Previous Data"
  Demux/2 -> Display2/1  "Slave Status"
  8 bytes concatinated converted to double/1 -> Gyroscope Int to Double Scale Factor/1  "gyr_x"
  Data Type Conversion/1 -> 8 bytes concatinated converted to double/1

== system DYC_controller/Hardware/SSIV Hardware Communication/gyr_y read message (Master --> Slave) ==
  Inport : Inport
  Mux : Mux
      settings: DisplayOption=signals
  Read Bit Set : simulink/Logic and Bit Operations/Bit Set  iBit=7
      settings: SourceProductName=Simulink  SourceProductBaseCode=SL
  uint8_t 1 : Constant  OutDataTypeStr=uint8
  uint8_t 2 : Constant  OutDataTypeStr=uint8
  uint8_t 3 : Constant  OutDataTypeStr=uint8
  Out1 : Outport
  wires:
  Read Bit Set/1 -> Mux/1  "Addres/RW Byte gyr_y Teensy Status will be returned here"
  uint8_t 1/1 -> Mux/2  "Junk will be returned here"
  Inport/1 -> Read Bit Set/1
  uint8_t 3/1 -> Mux/4  "Byte 1 will be returned here"
  Mux/1 -> Out1/1
  uint8_t 2/1 -> Mux/3  "Byte 0 will be returned here"

== system DYC_controller/Hardware/SSIV Hardware Communication/gyr_y return message (Slave --> Master) ==
  In1 : Inport
  8 bytes concatinated converted to double : DataTypeConversion  OutDataTypeStr=double  RndMeth=Nearest
  Bit Concat : hdlsllib/Logic and Bit Operations/Bit Concat  numInputs=2
      settings: SourceProductName=HDL Coder  SourceProductBaseCode=HD
  Bytes of the return message : Display
      settings: Format=decimal (Stored Integer)
  Data Type Conversion : DataTypeConversion  OutDataTypeStr=int16  RndMeth=Nearest
  Demux : Demux
  Display : Display
      settings: Format=binary (Stored Integer)
  Display1 : Display
      settings: Format=decimal (Stored Integer)
  Display2 : Display
      settings: Format=binary (Stored Integer)
  Gyroscope Int to Double Scale Factor : Gain  Gain=1/900
  gyr_y : Outport
  wires:
  8 bytes concatinated converted to double/1 -> Gyroscope Int to Double Scale Factor/1  "gyr_y"
  Demux/2 -> Display2/1  "Slave Status"
  Demux/1 -> Display/1  "Previous Data"
  In1/1 -> Bytes of the return message/1, Demux/1
  Bit Concat/1 -> Data Type Conversion/1
  Demux/4 -> Bit Concat/1
  Demux/3 -> Bit Concat/2
  Gyroscope Int to Double Scale Factor/1 -> Display1/1, gyr_y/1
  Data Type Conversion/1 -> 8 bytes concatinated converted to double/1
